simulink model "Problem_8"  (R2020a)
settings: Solver=VariableStepAuto  StartTime=0.0  StopTime=10.0  RelTol=1e-3
libraries: simulink x1
settings Model: Creator=intel  LastModifiedBy=Admin

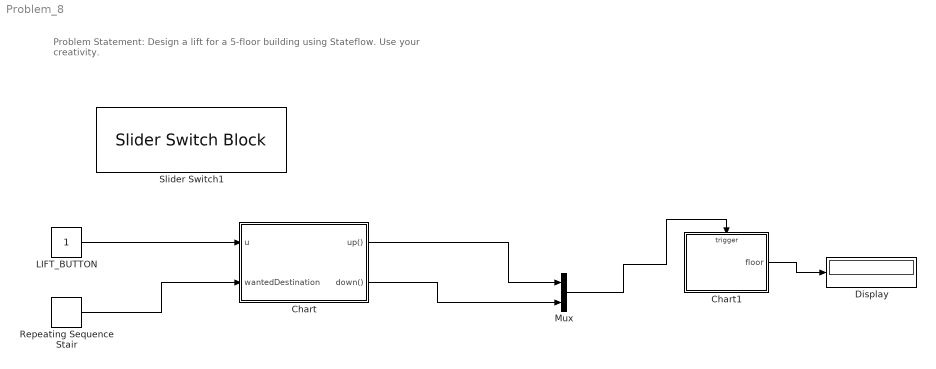
== system Problem_8 ==
  note: Problem Statement:
      | Design a lift for a 5-floor building using Stateflow. Use your creativity.
  Chart : Stateflow chart  TreatAsAtomicUnit=on
  Chart1 : Stateflow chart  TreatAsAtomicUnit=on
  Display : Display
  LIFT_BUTTON : Constant
  Mux : Mux  Inputs=2
  Repeating Sequence Stair : simulink/Sources/Repeating Sequence Stair  OutValues=[5 3 4 2 1].'  tsamp=-1  OutMin=[]  OutMax=[]  OutDataTypeStr=double  OutputDataTypeScalingMode=double  OutDataType=fixdt(0,8)  ConRadixGroup=Best Precision: Vector-wise  OutScaling=2^-12
  Slider Switch1 : SliderSwitchBlock
      settings: Values={{'UP', 'DOWN'}, [1 0]}
  wires:
  LIFT_BUTTON/1 -> Chart/1(u)
  Repeating Sequence Stair/1 -> Chart/2(wantedDestination)
  Chart/1(up()) -> Mux/1
  Mux/1 -> Chart1/Trigger
  Chart1/1(floor) -> Display/1
  Chart/2(down()) -> Mux/2

== stateflow chart Problem_8/Chart1 ==
  state ElevatorMoving
    state Floor_1
      entry:
      floor = 1;
    state Floor_2
      entry: floor = 2;
    state Floor_3
      en: floor = 3;
    state Floor_4
      en: floor = 4;
    state Floor_5
      en: floor = 5;
    (default) -> Floor_1
    Floor_2 -> Floor_1 [order 2] : up[wantedDestination<currentPosition]
    Floor_1 -> Floor_2 : down[wantedDestination>currentPosition]
    Floor_3 -> Floor_2 [order 2] : up[wantedDestination<currentPosition]
    Floor_2 -> Floor_3 [order 1] : down[wantedDestination>currentPosition]
    Floor_4 -> Floor_3 [order 1] : up
    Floor_3 -> Floor_4 [order 1] : down[wantedDestination>currentPosition]
    Floor_5 -> Floor_4 : up[wantedDestination<currentPosition]
    Floor_4 -> Floor_5 [order 2] : down[wantedDestination>currentPosition]
  data: floor output; wantedDestination local; currentPosition local
  events: down input RISING_EDGE_EVENT; up input RISING_EDGE_EVENT

== stateflow chart Problem_8/Chart ==
  state Controller_checking_for_user_inputs
  note: No_request
  state Preparing_to_Moving_Up
    state Door_Closing
      en:door=false;
    state Elevator_Starting
      en:currentPosition + 1;
    (default) -> Preparing_to_Moving_Up.Door_Closing
    Preparing_to_Moving_Up.Door_Closing -> Preparing_to_Moving_Up.Elevator_Starting
  state Preparing_to_Move_Down
    state Door_Closing
      en: door=false;
    state Elevator_Starting
      en:currentPosition = currentPosition - 1;
    (default) -> Preparing_to_Move_Down.Door_Closing
    Preparing_to_Move_Down.Door_Closing -> Preparing_to_Move_Down.Elevator_Starting
  state Elevator_System
    state elevator_moving
    state Elevator_Stopping
    state Elevator_Door_opening
    state Elevator_at_floor
    elevator_moving -> Elevator_Stopping : [currentPosition==wantedDestination]
    Elevator_Stopping -> Elevator_Door_opening : {door=true;}
    Elevator_Door_opening -> Elevator_at_floor
  note: ?
  state Elevator_Idle
  (default) -> Controller_checking_for_user_inputs
  Controller_checking_for_user_inputs -> (junction 56) [order 3]
  (junction 56) -> (junction 62)
  Controller_checking_for_user_inputs -> Preparing_to_Moving_Up.Door_Closing [order 1] : [u==1]
  Elevator_at_floor -> Controller_checking_for_user_inputs : Passenger_Exits
  Controller_checking_for_user_inputs -> Preparing_to_Move_Down.Door_Closing [order 2] : [u==0]
  Preparing_to_Moving_Up.Elevator_Starting -> Preparing_to_Moving_Up.Elevator_Starting : [wantedDestination<currentPosition]
  Preparing_to_Move_Down.Elevator_Starting -> Preparing_to_Move_Down.Elevator_Starting : [wantedDestination>currentPosition]
  (junction 37) -> Preparing_to_Moving_Up
  Preparing_to_Moving_Up -> elevator_moving : [wantedDestination<currentPosition]{up;}
  Elevator_Idle -> Preparing_to_Move_Down [order 2]
  Preparing_to_Move_Down -> elevator_moving : [wantedDestination>currentPosition]{down;}
  Elevator_Idle -> (junction 37) [order 1] : [currentPosition~=wantedDestination]
  (junction 62) -> Elevator_Idle
  data: u input; door local; wantedDestination input; currentPosition local
  events: up output FUNCTION_CALL_EVENT; down output FUNCTION_CALL_EVENT; Passenger_Exits local FUNCTION_CALL_EVENT
